simulink model "PID_simulink"  (R2013b)
settings: Solver=ode45  StartTime=0.0  StopTime=100  RelTol=1e-3
settings Model: Creator=Gert-Jan  LastModifiedBy=Gert-Jan

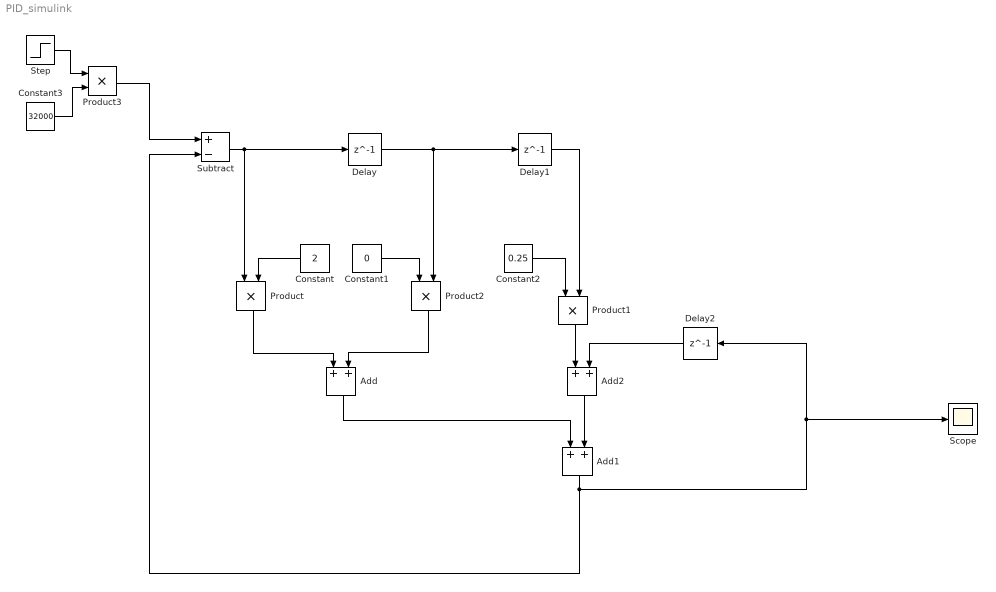
== system PID_simulink ==
  Add : Sum
  Add1 : Sum
  Add2 : Sum
  Constant : Constant  Value=2
  Constant1 : Constant  Value=0
  Constant2 : Constant  Value=0.25
  Constant3 : Constant  Value=32000
  Delay : Delay  DelayLength=1  SampleTime=1
  Delay1 : Delay  DelayLength=1  SampleTime=1
  Delay2 : Delay  DelayLength=1  SampleTime=1
  Product{,1..3} (4 alike) : Product
  Scope : Scope
  Step : Step  SampleTime=0
  Subtract : Sum  Inputs=+-
  wires:
  Subtract/1 -> Delay/1, Product/1
  Constant/1 -> Product/2
  Constant1/1 -> Product2/1
  Product2/1 -> Add/2
  Product/1 -> Add/1
  Add/1 -> Add1/1
  Add2/1 -> Add1/2
  Product1/1 -> Add2/1
  Constant2/1 -> Product1/1
  Add1/1 -> Scope/1, Delay2/1, Subtract/2
  Step/1 -> Product3/1
  Constant3/1 -> Product3/2
  Product3/1 -> Subtract/1
  Delay/1 -> Product2/2, Delay1/1
  Delay1/1 -> Product1/2
  Delay2/1 -> Add2/2
